simulink model "tank_sim"  (R2013a)
settings: Solver=ode45  StartTime=0.0  StopTime=10.0  RelTol=1e-3
values from neighbouring files (symbols this model uses):
  A = -Ao/Ai*k*g/sqrt(2*k*g*H0)    [konstante.m]
  Ai = 2    [konstante.m]
  Ao = 0.01    [konstante.m]
  B = 1/Ai    (= 0.5)    [konstante.m]
  C = [1]    [konstante.m]
  g = 9.81    [konstante.m]
  H0 = 5    [konstante.m]
  k = 1    [konstante.m]
  Q0 = Ao*sqrt(2*k*g*H0)    [konstante.m]
settings Model: Creator=Mirna  LastModifiedBy=Mirna

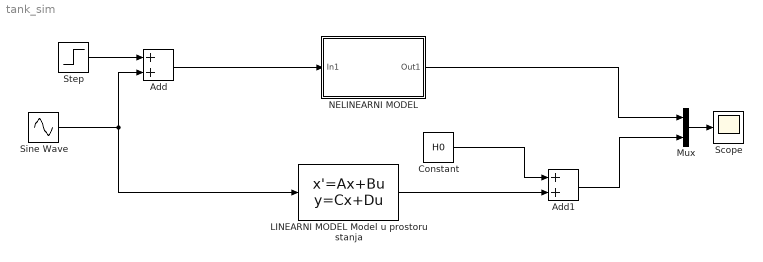
== system tank_sim ==
  Add : Sum
  Add1 : Sum
  Constant : Constant  Value=H0
  LINEARNI MODEL Model u prostoru stanja : StateSpace  A=A  B=B  C=C  D=[0]
  Mux : Mux  Inputs=2
  NELINEARNI MODEL : Subsystem
  Scope : Scope
  Sine Wave : Sin  Amplitude=0.1*Q0  Frequency=0.001*2*pi  SampleTime=0
  Step : Step  Time=0  After=Q0  SampleTime=0
  wires:
  Sine Wave/1 -> LINEARNI MODEL Model u prostoru stanja/1, Add/2
  Add/1 -> NELINEARNI MODEL/1(In1)
  LINEARNI MODEL Model u prostoru stanja/1 -> Add1/2
  Constant/1 -> Add1/1
  NELINEARNI MODEL/1(Out1) -> Mux/1
  Add1/1 -> Mux/2
  Mux/1 -> Scope/1
  Step/1 -> Add/1

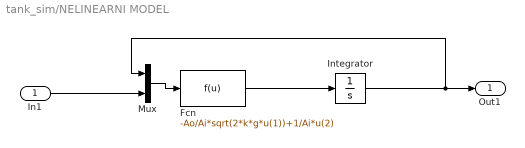
== system tank_sim/NELINEARNI MODEL ==
  In1 : Inport
  Fcn : Fcn  Expr=-Ao/Ai*sqrt(2*k*g*u(1))+1/Ai*u(2)
  Integrator : Integrator
  Mux : Mux  Inputs=2
  Out1 : Outport
  wires:
  Fcn/1 -> Integrator/1
  In1/1 -> Mux/2
  Mux/1 -> Fcn/1
  Integrator/1 -> Mux/1, Out1/1
